simulink library "myLib"  (R2023a)
settings: Solver=VariableStepAuto  StartTime=0.0  StopTime=10.0  RelTol=1e-3
settings Model: Creator=emcgarri  LastModifiedBy=emcgarri

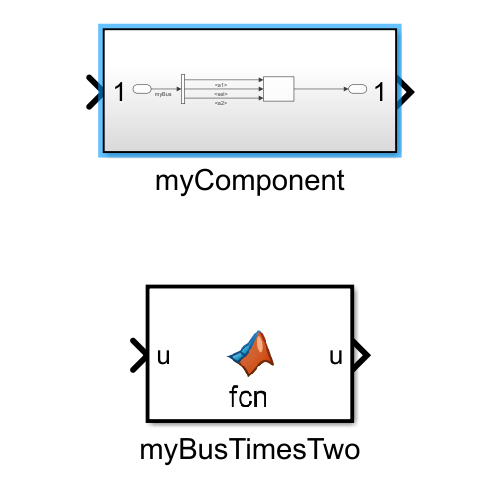
[thumbnail: Simulink's stored preview of the top-level diagram]
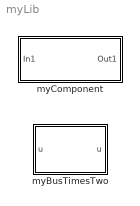
== system myLib ==
  myBusTimesTwo : MATLAB Function  TreatAsAtomicUnit=on
  myComponent : Subsystem

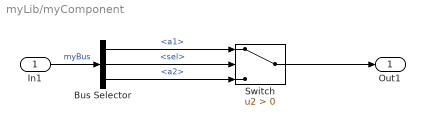
== system myLib/myComponent ==
  In1 : Inport  OutDataTypeStr=Bus: myBus
  Bus Selector : BusSelector  OutputSignals=a1,sel,a2
  Switch : Switch  Criteria=u2 > Threshold  SaturateOnIntegerOverflow=off  InputSameDT=off
  Out1 : Outport
  wires:
  In1/1 -> Bus Selector/1  "myBus"
  Bus Selector/2 -> Switch/2  "<sel>"
  Bus Selector/1 -> Switch/1  "<a1>"
  Bus Selector/3 -> Switch/3  "<a2>"
  Switch/1 -> Out1/1

== matlab function myLib/myBusTimesTwo ==
  data: u input Bus: myBus; u output
function u = fcn(u)
% Double the a1 and a2 fields
  u.a1 = u.a1 * 2;
  u.a2 = u.a2 * 2;
end
